simulink model "Control_planta_no_lineal_y_NN_mejor"  (R2023b)
settings: Solver=ode45  StartTime=0.0  StopTime=5000  RelTol=1e-3
values from neighbouring files (symbols this model uses):
  D = 0    [control_pid_tuning.m]
libraries: neural x98, simulink x9
(part 1 of 5)
settings Model: Creator=q  LastModifiedBy=q

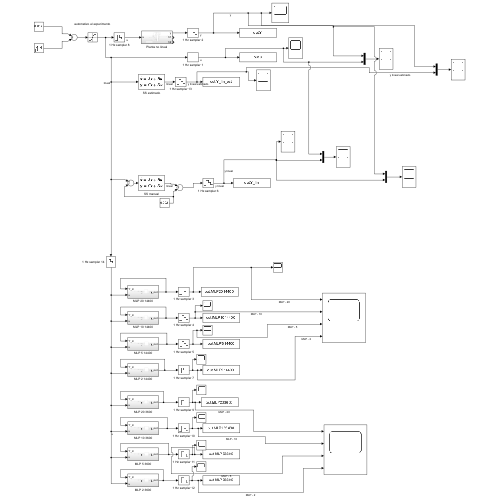
[thumbnail: Simulink's stored preview of the top-level diagram]
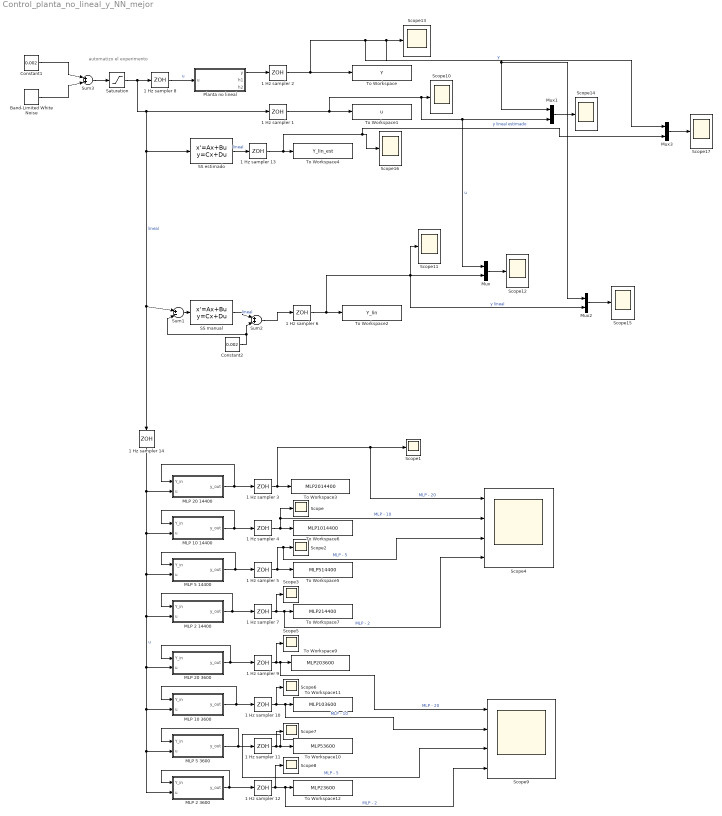
== system Control_planta_no_lineal_y_NN_mejor ==
  note: automatizo el experimento
  1 Hz sampler {1..14} (14 alike) : ZeroOrderHold
  Band-Limited White Noise : simulink/Sources/Band-Limited White Noise  Cov=[0.000002]  Ts=150  seed=[23341]
  Constant1 : Constant  Value=0.002
  Constant2 : Constant  Value=0.002
  MLP 10 14400 : Subsystem
  MLP 10 3600 : Subsystem
  MLP 2 14400 : Subsystem
  MLP 2 3600 : Subsystem
  MLP 20 14400 : Subsystem
  MLP 20 3600 : Subsystem
  MLP 5 14400 : Subsystem
  MLP 5 3600 : Subsystem
  Mux{,1..3} (4 alike) : Mux  Inputs=2
  Planta no lineal : Subsystem
  SS estimado : StateSpace  A=[-0.023375234759513,0.035713459182280;0.016442055191371,-0.031577082096728]  B=[2.537448139699421;-1.771387482474186]  C=[0.008723840649702,0.012539591066566]  D=0  InitialCondition=0
  SS manual : StateSpace  A=[-0.00359 0.000359;0.00976 -0.04878 ];  B=[2.92; 0]  C=[0 0.004905]  D=0  InitialCondition=0
  Saturation : Saturate  UpperLimit=0.0022  LowerLimit=0.0018
  Scope{,1..3,5..8,10..17} (16 alike) : Scope
  Scope4 : Scope  NumInputPorts=4
  Scope9 : Scope  NumInputPorts=4
  Sum1 : Sum  Inputs=|+-|
  Sum2 : Sum  Inputs=|++|
  Sum3 : Sum  Inputs=|++|
  To Workspace : ToWorkspace  VariableName=Y  SampleTime=1
  To Workspace1 : ToWorkspace  VariableName=u  SampleTime=1
  To Workspace10 : ToWorkspace  VariableName=MLP53600  SampleTime=1
  To Workspace11 : ToWorkspace  VariableName=MLP103600  SampleTime=1
  To Workspace12 : ToWorkspace  VariableName=MLP23600  SampleTime=1
  To Workspace2 : ToWorkspace  VariableName=Y_lin  SampleTime=1
  To Workspace3 : ToWorkspace  VariableName=MLP2014400  SampleTime=1
  To Workspace4 : ToWorkspace  VariableName=Y_lin_est  SampleTime=1
  To Workspace5 : ToWorkspace  VariableName=MLP514400  SampleTime=1
  To Workspace6 : ToWorkspace  VariableName=MLP1014400  SampleTime=1
  To Workspace7 : ToWorkspace  VariableName=MLP214400  SampleTime=1
  To Workspace9 : ToWorkspace  VariableName=MLP203600  SampleTime=1
  wires:
  Planta no lineal/1(y) -> 1 Hz sampler 2/1
  Constant1/1 -> Sum3/1
  Sum3/1 -> Saturation/1
  Band-Limited White Noise/1 -> Sum3/2
  1 Hz sampler 2/1 -> Mux3/1, Mux2/1, Mux1/1, Scope13/1, To Workspace/1  "y"
  1 Hz sampler 1/1 -> Mux1/2, Mux/1, Scope10/1, To Workspace1/1  "u"
  MLP 20 14400/1(y_out) -> 1 Hz sampler 3/1, MLP 20 14400/1(Y_in)
  1 Hz sampler 6/1 -> Mux/2, Mux2/2, Scope11/1, To Workspace2/1  "y lineal"
  MLP 10 14400/1(y_out) -> 1 Hz sampler 4/1, MLP 10 14400/1(Y_in)
  1 Hz sampler 3/1 -> Scope4/1, Scope1/1, To Workspace3/1  "MLP - 20"
  1 Hz sampler 4/1 -> Scope/1, Scope4/2, To Workspace6/1  "MLP - 10"
  1 Hz sampler 5/1 -> Scope4/3, Scope2/1, To Workspace5/1  "MLP - 5"
  MLP 5 14400/1(y_out) -> MLP 5 14400/1(Y_in), 1 Hz sampler 5/1
  MLP 2 14400/1(y_out) -> MLP 2 14400/1(Y_in), 1 Hz sampler 7/1
  1 Hz sampler 7/1 -> Scope4/4, To Workspace7/1, Scope3/1  "MLP - 2"
  1 Hz sampler 12/1 -> Scope9/4, To Workspace12/1, Scope8/1  "MLP - 2"
  MLP 2 3600/1(y_out) -> MLP 2 3600/1(Y_in), 1 Hz sampler 12/1
  MLP 5 3600/1(y_out) -> MLP 5 3600/1(Y_in), 1 Hz sampler 11/1
  1 Hz sampler 10/1 -> Scope9/2, To Workspace11/1, Scope6/1  "MLP - 10"
  1 Hz sampler 9/1 -> Scope5/1, Scope9/1, To Workspace9/1  "MLP - 20"
  MLP 10 3600/1(y_out) -> MLP 10 3600/1(Y_in), 1 Hz sampler 10/1
  MLP 20 3600/1(y_out) -> MLP 20 3600/1(Y_in), 1 Hz sampler 9/1
  1 Hz sampler 14/1 -> MLP 20 14400/2(u), MLP 10 14400/2(u), MLP 5 14400/2(u), MLP 2 14400/2(u), MLP 20 3600/2(u), MLP 10 3600/2(u), MLP 5 3600/2(u), MLP 2 3600/2(u)  "u"
  1 Hz sampler 11/1 -> Scope9/3, To Workspace10/1, Scope7/1  "MLP - 5"
  Mux/1 -> Scope12/1
  Mux1/1 -> Scope14/1
  1 Hz sampler 8/1 -> Planta no lineal/1(u)  "u"
  SS manual/1 -> Sum2/1  "lineal"
  Sum2/1 -> 1 Hz sampler 6/1
  Mux2/1 -> Scope15/1
  SS estimado/1 -> 1 Hz sampler 13/1  "lineal"
  1 Hz sampler 13/1 -> Mux3/2, Scope16/1, To Workspace4/1  "y lineal estimado"
  Mux3/1 -> Scope17/1
  Constant2/1 -> Sum1/2, Sum2/2
  Saturation/1 -> 1 Hz sampler 8/1, 1 Hz sampler 14/1, Sum1/1, SS estimado/1, 1 Hz sampler 1/1  "lineal"
  Sum1/1 -> SS manual/1

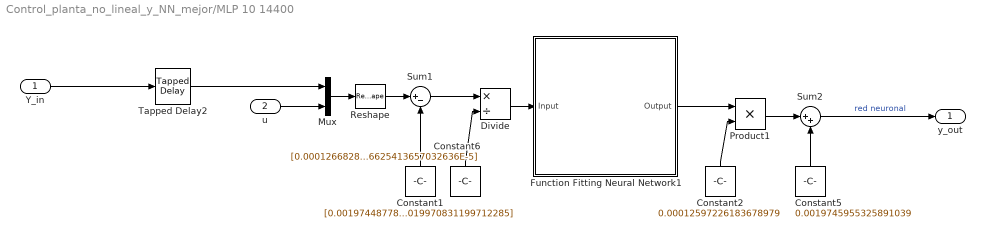
== system Control_planta_no_lineal_y_NN_mejor/MLP 10 14400 ==
  Y_in : Inport
  u : Inport  Port=2
  Constant1 : Constant  Value=[0.0019744877864955233 0.0019743785760481442 0.0019742678131102346 0.0019741553938777768 0.0019740411934791703 0.0019739250574736843 0.0019738067874396224 0.0019736861138403856 0.00197356263591298 0.001973435642133088 0.0019970831199712285]
  Constant2 : Constant  Value=0.00012597226183678979
  Constant5 : Constant  Value=0.0019745955325891039
  Constant6 : Constant  Value=[0.00012668289302772729 0.00012740789305343644 0.00012814838489358016 0.00012890570893586031 0.00012968150046382938 0.00013047781235730809 0.0001312973242993894 0.00013214373888773625 0.00013302266386210407 0.00013394425943220802 9.6625413657032636E-5]
  Divide : Product  Inputs=*/
  Function Fitting Neural Network1 : Subsystem
      mask help: Function Fitting Neural Network
      mask Display: e = 0.06;c1 = [120 150 230]/255;c2 = ([120 150 230]+0)/383;c3 = ([120 150 230]+128)/383;patch([0 1 1 0],[0 0 1 1],c1);patch([0 1 1 1-e 1-e 0+e],[0 0 1 1-e 0+e 0+e],c2);patch([0 0 1 1-e 0+e 0+e],[0 1 1 1-e 1-e 0+e],c3);plot([0 1 1 0 0],[0 0 1 1 0]);fprintf('NNET');port_label('input',1,' Input');port_label('output',1,'Output ');
  Mux : Mux  Inputs=2
  Product1 : Product
  Reshape : Reshape  OutputDimensionality=Column vector (2-D)
  Sum1 : Sum  Inputs=|+-
  Sum2 : Sum  Inputs=|++
  Tapped Delay2 : simulink/Discrete/Tapped Delay  vinit=0  samptime=1  NumDelays=10  DelayOrder=Newest  includeCurrent=off
  y_out : Outport
  wires:
  Sum2/1 -> y_out/1  "red neuronal"
  u/1 -> Mux/2
  Y_in/1 -> Tapped Delay2/1
  Sum1/1 -> Divide/1
  Constant2/1 -> Product1/2
  Product1/1 -> Sum2/1
  Constant5/1 -> Sum2/2
  Constant1/1 -> Sum1/2
  Constant6/1 -> Divide/2
  Tapped Delay2/1 -> Mux/1
  Mux/1 -> Reshape/1
  Reshape/1 -> Sum1/1
  Function Fitting Neural Network1/1(Output) -> Product1/1
  Divide/1 -> Function Fitting Neural Network1/1(Input)

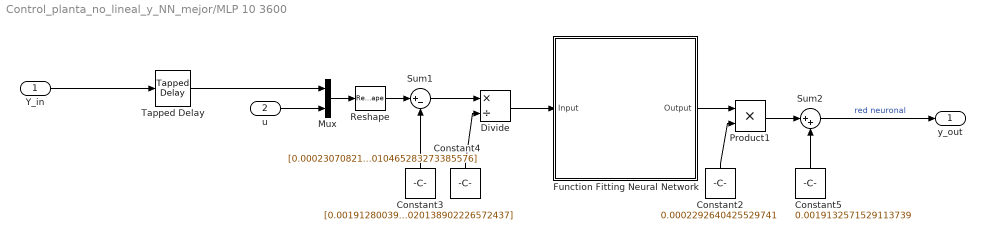
== system Control_planta_no_lineal_y_NN_mejor/MLP 10 3600 ==
  Y_in : Inport
  u : Inport  Port=2
  Constant2 : Constant  Value=0.0002292640425529741
  Constant3 : Constant  Value=[0.0019128003958595781 0.0019123379656579044 0.0019118695096077166 0.0019113946122121862 0.0019109127735299576 0.0019104233750979415 0.0019099256221635427 0.0019094184349221579 0.001908900207568905 0.0019083680886586006 0.0020138902226572437]
  Constant4 : Constant  Value=[0.00023070821663901105 0.00023218152875557362 0.00023368631301103448 0.00023522535857641475 0.00023680207245178661 0.00023842073740024686 0.00024008695208435038 0.00024180846512612068 0.00024359703442975925 0.00024547401204017618 0.00010465283273385576]
  Constant5 : Constant  Value=0.0019132571529113739
  Divide : Product  Inputs=*/
  Function Fitting Neural Network : Subsystem
      mask help: Function Fitting Neural Network
      mask Display: e = 0.06;c1 = [120 150 230]/255;c2 = ([120 150 230]+0)/383;c3 = ([120 150 230]+128)/383;patch([0 1 1 0],[0 0 1 1],c1);patch([0 1 1 1-e 1-e 0+e],[0 0 1 1-e 0+e 0+e],c2);patch([0 0 1 1-e 0+e 0+e],[0 1 1 1-e 1-e 0+e],c3);plot([0 1 1 0 0],[0 0 1 1 0]);fprintf('NNET');port_label('input',1,' Input');port_label('output',1,'Output ');
  Mux : Mux  Inputs=2
  Product1 : Product
  Reshape : Reshape  OutputDimensionality=Column vector (2-D)
  Sum1 : Sum  Inputs=|+-
  Sum2 : Sum  Inputs=|++
  Tapped Delay : simulink/Discrete/Tapped Delay  vinit=0  samptime=-1  NumDelays=10  DelayOrder=Newest  includeCurrent=off
  y_out : Outport
  wires:
  Constant4/1 -> Divide/2
  Mux/1 -> Reshape/1
  Tapped Delay/1 -> Mux/1
  Reshape/1 -> Sum1/1
  Product1/1 -> Sum2/1
  Sum2/1 -> y_out/1  "red neuronal"
  Constant5/1 -> Sum2/2
  Sum1/1 -> Divide/1
  u/1 -> Mux/2
  Constant2/1 -> Product1/2
  Constant3/1 -> Sum1/2
  Function Fitting Neural Network/1(Output) -> Product1/1
  Y_in/1 -> Tapped Delay/1
  Divide/1 -> Function Fitting Neural Network/1(Input)

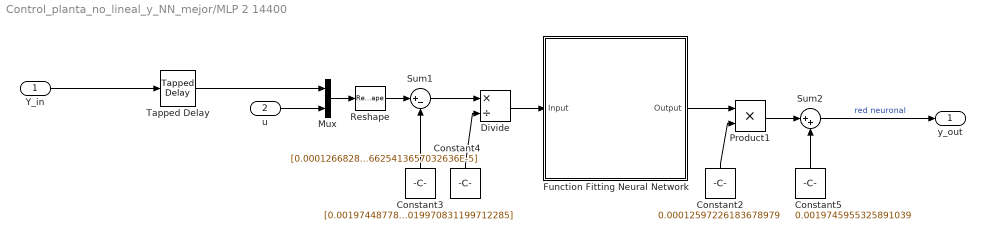
== system Control_planta_no_lineal_y_NN_mejor/MLP 2 14400 ==
  Y_in : Inport
  u : Inport  Port=2
  Constant2 : Constant  Value=0.00012597226183678979
  Constant3 : Constant  Value=[0.0019744877864955233 0.0019743785760481442 0.0019742678131102346 0.0019741553938777768 0.0019740411934791703 0.0019739250574736843 0.0019738067874396224 0.0019736861138403856 0.00197356263591298 0.001973435642133088 0.0019970831199712285]
  Constant4 : Constant  Value=[0.00012668289302772729 0.00012740789305343644 0.00012814838489358016 0.00012890570893586031 0.00012968150046382938 0.00013047781235730809 0.0001312973242993894 0.00013214373888773625 0.00013302266386210407 0.00013394425943220802 9.6625413657032636E-5]
  Constant5 : Constant  Value=0.0019745955325891039
  Divide : Product  Inputs=*/
  Function Fitting Neural Network : Subsystem
      mask help: Function Fitting Neural Network
      mask Display: e = 0.06;c1 = [120 150 230]/255;c2 = ([120 150 230]+0)/383;c3 = ([120 150 230]+128)/383;patch([0 1 1 0],[0 0 1 1],c1);patch([0 1 1 1-e 1-e 0+e],[0 0 1 1-e 0+e 0+e],c2);patch([0 0 1 1-e 0+e 0+e],[0 1 1 1-e 1-e 0+e],c3);plot([0 1 1 0 0],[0 0 1 1 0]);fprintf('NNET');port_label('input',1,' Input');port_label('output',1,'Output ');
  Mux : Mux  Inputs=2
  Product1 : Product
  Reshape : Reshape  OutputDimensionality=Column vector (2-D)
  Sum1 : Sum  Inputs=|+-
  Sum2 : Sum  Inputs=|++
  Tapped Delay : simulink/Discrete/Tapped Delay  vinit=0  samptime=-1  NumDelays=10  DelayOrder=Newest  includeCurrent=off
  y_out : Outport
  wires:
  Sum2/1 -> y_out/1  "red neuronal"
  u/1 -> Mux/2
  Y_in/1 -> Tapped Delay/1
  Sum1/1 -> Divide/1
  Constant2/1 -> Product1/2
  Product1/1 -> Sum2/1
  Constant5/1 -> Sum2/2
  Constant3/1 -> Sum1/2
  Constant4/1 -> Divide/2
  Mux/1 -> Reshape/1
  Reshape/1 -> Sum1/1
  Tapped Delay/1 -> Mux/1
  Divide/1 -> Function Fitting Neural Network/1(Input)
  Function Fitting Neural Network/1(Output) -> Product1/1

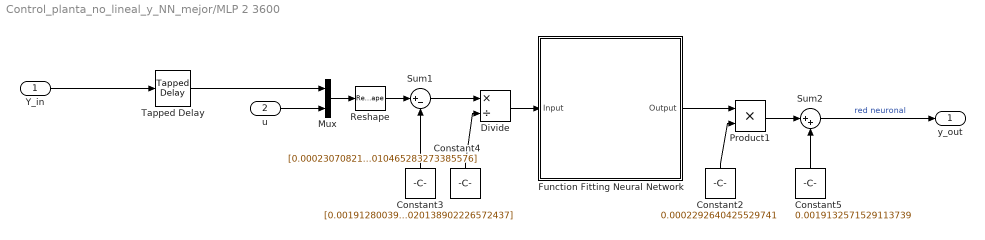
== system Control_planta_no_lineal_y_NN_mejor/MLP 2 3600 ==
  Y_in : Inport
  u : Inport  Port=2
  Constant2 : Constant  Value=0.0002292640425529741
  Constant3 : Constant  Value=[0.0019128003958595781 0.0019123379656579044 0.0019118695096077166 0.0019113946122121862 0.0019109127735299576 0.0019104233750979415 0.0019099256221635427 0.0019094184349221579 0.001908900207568905 0.0019083680886586006 0.0020138902226572437]
  Constant4 : Constant  Value=[0.00023070821663901105 0.00023218152875557362 0.00023368631301103448 0.00023522535857641475 0.00023680207245178661 0.00023842073740024686 0.00024008695208435038 0.00024180846512612068 0.00024359703442975925 0.00024547401204017618 0.00010465283273385576]
  Constant5 : Constant  Value=0.0019132571529113739
  Divide : Product  Inputs=*/
  Function Fitting Neural Network : Subsystem
      mask help: Function Fitting Neural Network
      mask Display: e = 0.06;c1 = [120 150 230]/255;c2 = ([120 150 230]+0)/383;c3 = ([120 150 230]+128)/383;patch([0 1 1 0],[0 0 1 1],c1);patch([0 1 1 1-e 1-e 0+e],[0 0 1 1-e 0+e 0+e],c2);patch([0 0 1 1-e 0+e 0+e],[0 1 1 1-e 1-e 0+e],c3);plot([0 1 1 0 0],[0 0 1 1 0]);fprintf('NNET');port_label('input',1,' Input');port_label('output',1,'Output ');
  Mux : Mux  Inputs=2
  Product1 : Product
  Reshape : Reshape  OutputDimensionality=Column vector (2-D)
  Sum1 : Sum  Inputs=|+-
  Sum2 : Sum  Inputs=|++
  Tapped Delay : simulink/Discrete/Tapped Delay  vinit=0  samptime=-1  NumDelays=10  DelayOrder=Newest  includeCurrent=off
  y_out : Outport
  wires:
  Constant4/1 -> Divide/2
  Mux/1 -> Reshape/1
  Tapped Delay/1 -> Mux/1
  Reshape/1 -> Sum1/1
  Product1/1 -> Sum2/1
  Sum2/1 -> y_out/1  "red neuronal"
  Constant5/1 -> Sum2/2
  Sum1/1 -> Divide/1
  u/1 -> Mux/2
  Constant2/1 -> Product1/2
  Constant3/1 -> Sum1/2
  Function Fitting Neural Network/1(Output) -> Product1/1
  Y_in/1 -> Tapped Delay/1
  Divide/1 -> Function Fitting Neural Network/1(Input)

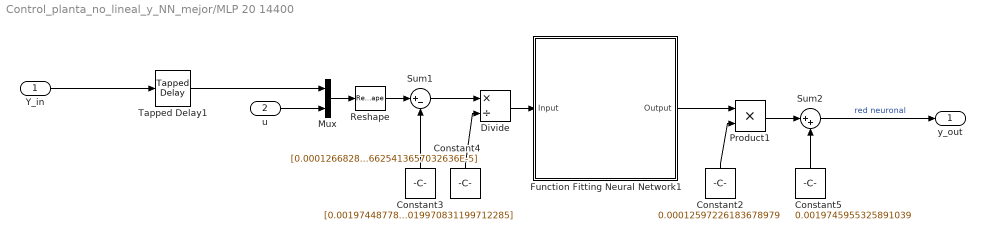
== system Control_planta_no_lineal_y_NN_mejor/MLP 20 14400 ==
  Y_in : Inport
  u : Inport  Port=2
  Constant2 : Constant  Value=0.00012597226183678979
  Constant3 : Constant  Value=[0.0019744877864955233 0.0019743785760481442 0.0019742678131102346 0.0019741553938777768 0.0019740411934791703 0.0019739250574736843 0.0019738067874396224 0.0019736861138403856 0.00197356263591298 0.001973435642133088 0.0019970831199712285]
  Constant4 : Constant  Value=[0.00012668289302772729 0.00012740789305343644 0.00012814838489358016 0.00012890570893586031 0.00012968150046382938 0.00013047781235730809 0.0001312973242993894 0.00013214373888773625 0.00013302266386210407 0.00013394425943220802 9.6625413657032636E-5]
  Constant5 : Constant  Value=0.0019745955325891039
  Divide : Product  Inputs=*/
  Function Fitting Neural Network1 : Subsystem
      mask help: Function Fitting Neural Network
      mask Display: e = 0.06;c1 = [120 150 230]/255;c2 = ([120 150 230]+0)/383;c3 = ([120 150 230]+128)/383;patch([0 1 1 0],[0 0 1 1],c1);patch([0 1 1 1-e 1-e 0+e],[0 0 1 1-e 0+e 0+e],c2);patch([0 0 1 1-e 0+e 0+e],[0 1 1 1-e 1-e 0+e],c3);plot([0 1 1 0 0],[0 0 1 1 0]);fprintf('NNET');port_label('input',1,' Input');port_label('output',1,'Output ');
  Mux : Mux  Inputs=2
  Product1 : Product
  Reshape : Reshape  OutputDimensionality=Column vector (2-D)
  Sum1 : Sum  Inputs=|+-
  Sum2 : Sum  Inputs=|++
  Tapped Delay1 : simulink/Discrete/Tapped Delay  vinit=0  samptime=1  NumDelays=10  DelayOrder=Newest  includeCurrent=off
  y_out : Outport
  wires:
  Constant3/1 -> Sum1/2
  Constant4/1 -> Divide/2
  Mux/1 -> Reshape/1
  Tapped Delay1/1 -> Mux/1
  Sum1/1 -> Divide/1
  Constant5/1 -> Sum2/2
  Reshape/1 -> Sum1/1
  Product1/1 -> Sum2/1
  Constant2/1 -> Product1/2
  Y_in/1 -> Tapped Delay1/1
  u/1 -> Mux/2
  Sum2/1 -> y_out/1  "red neuronal"
  Divide/1 -> Function Fitting Neural Network1/1(Input)
  Function Fitting Neural Network1/1(Output) -> Product1/1

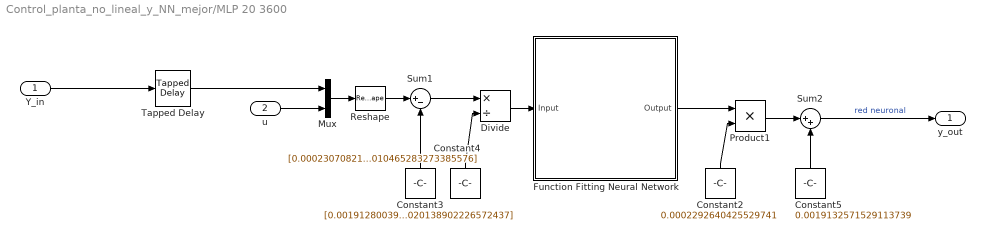
== system Control_planta_no_lineal_y_NN_mejor/MLP 20 3600 ==
  Y_in : Inport
  u : Inport  Port=2
  Constant2 : Constant  Value=0.0002292640425529741
  Constant3 : Constant  Value=[0.0019128003958595781 0.0019123379656579044 0.0019118695096077166 0.0019113946122121862 0.0019109127735299576 0.0019104233750979415 0.0019099256221635427 0.0019094184349221579 0.001908900207568905 0.0019083680886586006 0.0020138902226572437]
  Constant4 : Constant  Value=[0.00023070821663901105 0.00023218152875557362 0.00023368631301103448 0.00023522535857641475 0.00023680207245178661 0.00023842073740024686 0.00024008695208435038 0.00024180846512612068 0.00024359703442975925 0.00024547401204017618 0.00010465283273385576]
  Constant5 : Constant  Value=0.0019132571529113739
  Divide : Product  Inputs=*/
  Function Fitting Neural Network : Subsystem
      mask help: Function Fitting Neural Network
      mask Display: e = 0.06;c1 = [120 150 230]/255;c2 = ([120 150 230]+0)/383;c3 = ([120 150 230]+128)/383;patch([0 1 1 0],[0 0 1 1],c1);patch([0 1 1 1-e 1-e 0+e],[0 0 1 1-e 0+e 0+e],c2);patch([0 0 1 1-e 0+e 0+e],[0 1 1 1-e 1-e 0+e],c3);plot([0 1 1 0 0],[0 0 1 1 0]);fprintf('NNET');port_label('input',1,' Input');port_label('output',1,'Output ');
  Mux : Mux  Inputs=2
  Product1 : Product
  Reshape : Reshape  OutputDimensionality=Column vector (2-D)
  Sum1 : Sum  Inputs=|+-
  Sum2 : Sum  Inputs=|++
  Tapped Delay : simulink/Discrete/Tapped Delay  vinit=0  samptime=-1  NumDelays=10  DelayOrder=Newest  includeCurrent=off
  y_out : Outport
  wires:
  Sum2/1 -> y_out/1  "red neuronal"
  u/1 -> Mux/2
  Y_in/1 -> Tapped Delay/1
  Sum1/1 -> Divide/1
  Constant2/1 -> Product1/2
  Product1/1 -> Sum2/1
  Constant5/1 -> Sum2/2
  Constant3/1 -> Sum1/2
  Constant4/1 -> Divide/2
  Tapped Delay/1 -> Mux/1
  Mux/1 -> Reshape/1
  Reshape/1 -> Sum1/1
  Function Fitting Neural Network/1(Output) -> Product1/1
  Divide/1 -> Function Fitting Neural Network/1(Input)

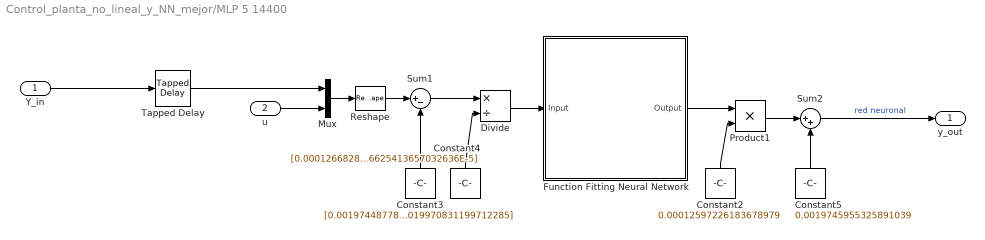
== system Control_planta_no_lineal_y_NN_mejor/MLP 5 14400 ==
  Y_in : Inport
  u : Inport  Port=2
  Constant2 : Constant  Value=0.00012597226183678979
  Constant3 : Constant  Value=[0.0019744877864955233 0.0019743785760481442 0.0019742678131102346 0.0019741553938777768 0.0019740411934791703 0.0019739250574736843 0.0019738067874396224 0.0019736861138403856 0.00197356263591298 0.001973435642133088 0.0019970831199712285]
  Constant4 : Constant  Value=[0.00012668289302772729 0.00012740789305343644 0.00012814838489358016 0.00012890570893586031 0.00012968150046382938 0.00013047781235730809 0.0001312973242993894 0.00013214373888773625 0.00013302266386210407 0.00013394425943220802 9.6625413657032636E-5]
  Constant5 : Constant  Value=0.0019745955325891039
  Divide : Product  Inputs=*/
  Function Fitting Neural Network : Subsystem
      mask help: Function Fitting Neural Network
      mask Display: e = 0.06;c1 = [120 150 230]/255;c2 = ([120 150 230]+0)/383;c3 = ([120 150 230]+128)/383;patch([0 1 1 0],[0 0 1 1],c1);patch([0 1 1 1-e 1-e 0+e],[0 0 1 1-e 0+e 0+e],c2);patch([0 0 1 1-e 0+e 0+e],[0 1 1 1-e 1-e 0+e],c3);plot([0 1 1 0 0],[0 0 1 1 0]);fprintf('NNET');port_label('input',1,' Input');port_label('output',1,'Output ');
  Mux : Mux  Inputs=2
  Product1 : Product
  Reshape : Reshape  OutputDimensionality=Column vector (2-D)
  Sum1 : Sum  Inputs=|+-
  Sum2 : Sum  Inputs=|++
  Tapped Delay : simulink/Discrete/Tapped Delay  vinit=0  samptime=-1  NumDelays=10  DelayOrder=Newest  includeCurrent=off
  y_out : Outport
  wires:
  Sum2/1 -> y_out/1  "red neuronal"
  u/1 -> Mux/2
  Y_in/1 -> Tapped Delay/1
  Sum1/1 -> Divide/1
  Constant2/1 -> Product1/2
  Product1/1 -> Sum2/1
  Constant5/1 -> Sum2/2
  Constant3/1 -> Sum1/2
  Constant4/1 -> Divide/2
  Tapped Delay/1 -> Mux/1
  Mux/1 -> Reshape/1
  Reshape/1 -> Sum1/1
  Divide/1 -> Function Fitting Neural Network/1(Input)
  Function Fitting Neural Network/1(Output) -> Product1/1

== system Control_planta_no_lineal_y_NN_mejor/MLP 5 3600 ==
  Y_in : Inport
  u : Inport  Port=2
  Constant2 : Constant  Value=0.0002292640425529741
  Constant3 : Constant  Value=[0.0019128003958595781 0.0019123379656579044 0.0019118695096077166 0.0019113946122121862 0.0019109127735299576 0.0019104233750979415 0.0019099256221635427 0.0019094184349221579 0.001908900207568905 0.0019083680886586006 0.0020138902226572437]
  Constant4 : Constant  Value=[0.00023070821663901105 0.00023218152875557362 0.00023368631301103448 0.00023522535857641475 0.00023680207245178661 0.00023842073740024686 0.00024008695208435038 0.00024180846512612068 0.00024359703442975925 0.00024547401204017618 0.00010465283273385576]
  Constant5 : Constant  Value=0.0019132571529113739
  Divide : Product  Inputs=*/
  Function Fitting Neural Network : Subsystem
      mask help: Function Fitting Neural Network
      mask Display: e = 0.06;c1 = [120 150 230]/255;c2 = ([120 150 230]+0)/383;c3 = ([120 150 230]+128)/383;patch([0 1 1 0],[0 0 1 1],c1);patch([0 1 1 1-e 1-e 0+e],[0 0 1 1-e 0+e 0+e],c2);patch([0 0 1 1-e 0+e 0+e],[0 1 1 1-e 1-e 0+e],c3);plot([0 1 1 0 0],[0 0 1 1 0]);fprintf('NNET');port_label('input',1,' Input');port_label('output',1,'Output ');
  Mux : Mux  Inputs=2
  Product1 : Product
  Reshape : Reshape  OutputDimensionality=Column vector (2-D)
  Sum1 : Sum  Inputs=|+-
  Sum2 : Sum  Inputs=|++
  Tapped Delay : simulink/Discrete/Tapped Delay  vinit=0  samptime=-1  NumDelays=10  DelayOrder=Newest  includeCurrent=off
  y_out : Outport
  wires:
  Constant4/1 -> Divide/2
  Mux/1 -> Reshape/1
  Tapped Delay/1 -> Mux/1
  Reshape/1 -> Sum1/1
  Product1/1 -> Sum2/1
  Sum2/1 -> y_out/1  "red neuronal"
  Constant5/1 -> Sum2/2
  Sum1/1 -> Divide/1
  u/1 -> Mux/2
  Constant2/1 -> Product1/2
  Constant3/1 -> Sum1/2
  Y_in/1 -> Tapped Delay/1
  Divide/1 -> Function Fitting Neural Network/1(Input)
  Function Fitting Neural Network/1(Output) -> Product1/1

== system Control_planta_no_lineal_y_NN_mejor/Planta no lineal ==
  note: A1 =0.342   m²   (tanque 1 ≈ 66 cm de diámetro)
      | A2 = 0.126   m²   (tanque 2 ≈ 40 cm diámetro)
  u : Inport
  A1 : Constant  Value=0.342119439975929
  A2 : Constant  Value=0.125663706143592
  Constant1 : Constant  Value=0
  Constant6 : Constant  Value=0
  Integrator1 : Integrator  InitialConditionSource=external
  Integrator2 : Integrator  InitialConditionSource=external
  K12 : Constant  Value=5e-4
  K2 : Constant  Value=1e-3
  MATLAB Function : MATLAB Function  TreatAsAtomicUnit=on
  y : Outport
  h1 : Outport  Port=2
  h2 : Outport  Port=3
  wires:
  K2/1 -> MATLAB Function/5(k2)
  MATLAB Function/3(dh2) -> Integrator2/1
  MATLAB Function/2(dh1) -> Integrator1/1
  Integrator1/1 -> h1/1, MATLAB Function/1(h1)
  Constant6/1 -> Integrator2/2
  A2/1 -> MATLAB Function/7(A2)
  Constant1/1 -> Integrator1/2
  u/1 -> MATLAB Function/3(u)
  MATLAB Function/1(y) -> y/1
  Integrator2/1 -> h2/1, MATLAB Function/2(h2)
  A1/1 -> MATLAB Function/6(A1)
  K12/1 -> MATLAB Function/4(k12)

== system Control_planta_no_lineal_y_NN_mejor/MLP 10 14400/Function Fitting Neural Network1 ==
  Input : Inport  PortDimensions=11
      mask Display: e = 0.06;c1 = [120 230 180]/255;c2 = ([120 230 180]+0)/(256+128);c3 = ([120 230 180]+128)/(256+128);patch([0 1 1 0],[0 0 1 1],c1);patch([0 1 1 1-e 1-e 0+e],[0 0 1 1-e 0+e 0+e],c2);patch([0 0 1 1-e 0+e 0+e],[0 1 1 1-e 1-e 0+e],c3);plot([0 1 1 0 0],[0 0 1 1 0]);
  Layer 1 : Subsystem
      mask Display: e = 0.06;c1 = [120 150 230]/255;c2 = ([120 150 230]+0)/383;c3 = ([120 150 230]+128)/383;patch([0 1 1 0],[0 0 1 1],c1);patch([0 1 1 1-e 1-e 0+e],[0 0 1 1-e 0+e 0+e],c2);patch([0 0 1 1-e 0+e 0+e],[0 1 1 1-e 1-e 0+e],c3);plot([0 1 1 0 0],[0 0 1 1 0]);
  Layer 2 : Subsystem
      mask Display: e = 0.06;c1 = [120 150 230]/255;c2 = ([120 150 230]+0)/383;c3 = ([120 150 230]+128)/383;patch([0 1 1 0],[0 0 1 1],c1);patch([0 1 1 1-e 1-e 0+e],[0 0 1 1-e 0+e 0+e],c2);patch([0 0 1 1-e 0+e 0+e],[0 1 1 1-e 1-e 0+e],c3);plot([0 1 1 0 0],[0 0 1 1 0]);
  Process Input 1 : Subsystem
      mask Display: e = 0.06;c1 = [120 150 230]/255;c2 = ([120 150 230]+0)/383;c3 = ([120 150 230]+128)/383;patch([0 1 1 0],[0 0 1 1],c1);patch([0 1 1 1-e 1-e 0+e],[0 0 1 1-e 0+e 0+e],c2);patch([0 0 1 1-e 0+e 0+e],[0 1 1 1-e 1-e 0+e],c3);plot([0 1 1 0 0],[0 0 1 1 0]);
  Process Output 1 : Subsystem
      mask Display: e = 0.06;c1 = [120 150 230]/255;c2 = ([120 150 230]+0)/383;c3 = ([120 150 230]+128)/383;patch([0 1 1 0],[0 0 1 1],c1);patch([0 1 1 1-e 1-e 0+e],[0 0 1 1-e 0+e 0+e],c2);patch([0 0 1 1-e 0+e 0+e],[0 1 1 1-e 1-e 0+e],c3);plot([0 1 1 0 0],[0 0 1 1 0]);
  Output : Outport  InitialOutput=0
      mask Display: e = 0.06;c1 = [120 230 180]/255;c2 = ([120 230 180]+0)/(256+128);c3 = ([120 230 180]+128)/(256+128);patch([0 1 1 0],[0 0 1 1],c1);patch([0 1 1 1-e 1-e 0+e],[0 0 1 1-e 0+e 0+e],c2);patch([0 0 1 1-e 0+e 0+e],[0 1 1 1-e 1-e 0+e],c3);plot([0 1 1 0 0],[0 0 1 1 0]);
  wires:
  Input/1 -> Process Input 1/1(x)
  Process Output 1/1(y) -> Output/1
  Process Input 1/1(p) -> Layer 1/1("p{1}")
  Layer 1/1("a{1}") -> [feedback1]
  [feedback1] -> Layer 2/1("a{1} ")
  Layer 2/1("a{2}") -> Process Output 1/1(a)

== system Control_planta_no_lineal_y_NN_mejor/MLP 10 3600/Function Fitting Neural Network ==
  Input : Inport  PortDimensions=11
      mask Display: e = 0.06;c1 = [120 230 180]/255;c2 = ([120 230 180]+0)/(256+128);c3 = ([120 230 180]+128)/(256+128);patch([0 1 1 0],[0 0 1 1],c1);patch([0 1 1 1-e 1-e 0+e],[0 0 1 1-e 0+e 0+e],c2);patch([0 0 1 1-e 0+e 0+e],[0 1 1 1-e 1-e 0+e],c3);plot([0 1 1 0 0],[0 0 1 1 0]);
  Layer 1 : Subsystem
      mask Display: e = 0.06;c1 = [120 150 230]/255;c2 = ([120 150 230]+0)/383;c3 = ([120 150 230]+128)/383;patch([0 1 1 0],[0 0 1 1],c1);patch([0 1 1 1-e 1-e 0+e],[0 0 1 1-e 0+e 0+e],c2);patch([0 0 1 1-e 0+e 0+e],[0 1 1 1-e 1-e 0+e],c3);plot([0 1 1 0 0],[0 0 1 1 0]);
  Layer 2 : Subsystem
      mask Display: e = 0.06;c1 = [120 150 230]/255;c2 = ([120 150 230]+0)/383;c3 = ([120 150 230]+128)/383;patch([0 1 1 0],[0 0 1 1],c1);patch([0 1 1 1-e 1-e 0+e],[0 0 1 1-e 0+e 0+e],c2);patch([0 0 1 1-e 0+e 0+e],[0 1 1 1-e 1-e 0+e],c3);plot([0 1 1 0 0],[0 0 1 1 0]);
  Process Input 1 : Subsystem
      mask Display: e = 0.06;c1 = [120 150 230]/255;c2 = ([120 150 230]+0)/383;c3 = ([120 150 230]+128)/383;patch([0 1 1 0],[0 0 1 1],c1);patch([0 1 1 1-e 1-e 0+e],[0 0 1 1-e 0+e 0+e],c2);patch([0 0 1 1-e 0+e 0+e],[0 1 1 1-e 1-e 0+e],c3);plot([0 1 1 0 0],[0 0 1 1 0]);
  Process Output 1 : Subsystem
      mask Display: e = 0.06;c1 = [120 150 230]/255;c2 = ([120 150 230]+0)/383;c3 = ([120 150 230]+128)/383;patch([0 1 1 0],[0 0 1 1],c1);patch([0 1 1 1-e 1-e 0+e],[0 0 1 1-e 0+e 0+e],c2);patch([0 0 1 1-e 0+e 0+e],[0 1 1 1-e 1-e 0+e],c3);plot([0 1 1 0 0],[0 0 1 1 0]);
  Output : Outport  InitialOutput=0
      mask Display: e = 0.06;c1 = [120 230 180]/255;c2 = ([120 230 180]+0)/(256+128);c3 = ([120 230 180]+128)/(256+128);patch([0 1 1 0],[0 0 1 1],c1);patch([0 1 1 1-e 1-e 0+e],[0 0 1 1-e 0+e 0+e],c2);patch([0 0 1 1-e 0+e 0+e],[0 1 1 1-e 1-e 0+e],c3);plot([0 1 1 0 0],[0 0 1 1 0]);
  wires:
  Input/1 -> Process Input 1/1(x)
  Process Output 1/1(y) -> Output/1
  Process Input 1/1(p) -> Layer 1/1("p{1}")
  Layer 1/1("a{1}") -> [feedback1]
  [feedback1] -> Layer 2/1("a{1} ")
  Layer 2/1("a{2}") -> Process Output 1/1(a)

== system Control_planta_no_lineal_y_NN_mejor/MLP 2 14400/Function Fitting Neural Network ==
  Input : Inport  PortDimensions=11
      mask Display: e = 0.06;c1 = [120 230 180]/255;c2 = ([120 230 180]+0)/(256+128);c3 = ([120 230 180]+128)/(256+128);patch([0 1 1 0],[0 0 1 1],c1);patch([0 1 1 1-e 1-e 0+e],[0 0 1 1-e 0+e 0+e],c2);patch([0 0 1 1-e 0+e 0+e],[0 1 1 1-e 1-e 0+e],c3);plot([0 1 1 0 0],[0 0 1 1 0]);
  Layer 1 : Subsystem
      mask Display: e = 0.06;c1 = [120 150 230]/255;c2 = ([120 150 230]+0)/383;c3 = ([120 150 230]+128)/383;patch([0 1 1 0],[0 0 1 1],c1);patch([0 1 1 1-e 1-e 0+e],[0 0 1 1-e 0+e 0+e],c2);patch([0 0 1 1-e 0+e 0+e],[0 1 1 1-e 1-e 0+e],c3);plot([0 1 1 0 0],[0 0 1 1 0]);
  Layer 2 : Subsystem
      mask Display: e = 0.06;c1 = [120 150 230]/255;c2 = ([120 150 230]+0)/383;c3 = ([120 150 230]+128)/383;patch([0 1 1 0],[0 0 1 1],c1);patch([0 1 1 1-e 1-e 0+e],[0 0 1 1-e 0+e 0+e],c2);patch([0 0 1 1-e 0+e 0+e],[0 1 1 1-e 1-e 0+e],c3);plot([0 1 1 0 0],[0 0 1 1 0]);
  Process Input 1 : Subsystem
      mask Display: e = 0.06;c1 = [120 150 230]/255;c2 = ([120 150 230]+0)/383;c3 = ([120 150 230]+128)/383;patch([0 1 1 0],[0 0 1 1],c1);patch([0 1 1 1-e 1-e 0+e],[0 0 1 1-e 0+e 0+e],c2);patch([0 0 1 1-e 0+e 0+e],[0 1 1 1-e 1-e 0+e],c3);plot([0 1 1 0 0],[0 0 1 1 0]);
  Process Output 1 : Subsystem
      mask Display: e = 0.06;c1 = [120 150 230]/255;c2 = ([120 150 230]+0)/383;c3 = ([120 150 230]+128)/383;patch([0 1 1 0],[0 0 1 1],c1);patch([0 1 1 1-e 1-e 0+e],[0 0 1 1-e 0+e 0+e],c2);patch([0 0 1 1-e 0+e 0+e],[0 1 1 1-e 1-e 0+e],c3);plot([0 1 1 0 0],[0 0 1 1 0]);
  Output : Outport  InitialOutput=0
      mask Display: e = 0.06;c1 = [120 230 180]/255;c2 = ([120 230 180]+0)/(256+128);c3 = ([120 230 180]+128)/(256+128);patch([0 1 1 0],[0 0 1 1],c1);patch([0 1 1 1-e 1-e 0+e],[0 0 1 1-e 0+e 0+e],c2);patch([0 0 1 1-e 0+e 0+e],[0 1 1 1-e 1-e 0+e],c3);plot([0 1 1 0 0],[0 0 1 1 0]);
  wires:
  Input/1 -> Process Input 1/1(x)
  Process Output 1/1(y) -> Output/1
  Process Input 1/1(p) -> Layer 1/1("p{1}")
  Layer 1/1("a{1}") -> [feedback1]
  [feedback1] -> Layer 2/1("a{1} ")
  Layer 2/1("a{2}") -> Process Output 1/1(a)

== system Control_planta_no_lineal_y_NN_mejor/MLP 2 3600/Function Fitting Neural Network ==
  Input : Inport  PortDimensions=11
      mask Display: e = 0.06;c1 = [120 230 180]/255;c2 = ([120 230 180]+0)/(256+128);c3 = ([120 230 180]+128)/(256+128);patch([0 1 1 0],[0 0 1 1],c1);patch([0 1 1 1-e 1-e 0+e],[0 0 1 1-e 0+e 0+e],c2);patch([0 0 1 1-e 0+e 0+e],[0 1 1 1-e 1-e 0+e],c3);plot([0 1 1 0 0],[0 0 1 1 0]);
  Layer 1 : Subsystem
      mask Display: e = 0.06;c1 = [120 150 230]/255;c2 = ([120 150 230]+0)/383;c3 = ([120 150 230]+128)/383;patch([0 1 1 0],[0 0 1 1],c1);patch([0 1 1 1-e 1-e 0+e],[0 0 1 1-e 0+e 0+e],c2);patch([0 0 1 1-e 0+e 0+e],[0 1 1 1-e 1-e 0+e],c3);plot([0 1 1 0 0],[0 0 1 1 0]);
  Layer 2 : Subsystem
      mask Display: e = 0.06;c1 = [120 150 230]/255;c2 = ([120 150 230]+0)/383;c3 = ([120 150 230]+128)/383;patch([0 1 1 0],[0 0 1 1],c1);patch([0 1 1 1-e 1-e 0+e],[0 0 1 1-e 0+e 0+e],c2);patch([0 0 1 1-e 0+e 0+e],[0 1 1 1-e 1-e 0+e],c3);plot([0 1 1 0 0],[0 0 1 1 0]);
  Process Input 1 : Subsystem
      mask Display: e = 0.06;c1 = [120 150 230]/255;c2 = ([120 150 230]+0)/383;c3 = ([120 150 230]+128)/383;patch([0 1 1 0],[0 0 1 1],c1);patch([0 1 1 1-e 1-e 0+e],[0 0 1 1-e 0+e 0+e],c2);patch([0 0 1 1-e 0+e 0+e],[0 1 1 1-e 1-e 0+e],c3);plot([0 1 1 0 0],[0 0 1 1 0]);
  Process Output 1 : Subsystem
      mask Display: e = 0.06;c1 = [120 150 230]/255;c2 = ([120 150 230]+0)/383;c3 = ([120 150 230]+128)/383;patch([0 1 1 0],[0 0 1 1],c1);patch([0 1 1 1-e 1-e 0+e],[0 0 1 1-e 0+e 0+e],c2);patch([0 0 1 1-e 0+e 0+e],[0 1 1 1-e 1-e 0+e],c3);plot([0 1 1 0 0],[0 0 1 1 0]);
  Output : Outport  InitialOutput=0
      mask Display: e = 0.06;c1 = [120 230 180]/255;c2 = ([120 230 180]+0)/(256+128);c3 = ([120 230 180]+128)/(256+128);patch([0 1 1 0],[0 0 1 1],c1);patch([0 1 1 1-e 1-e 0+e],[0 0 1 1-e 0+e 0+e],c2);patch([0 0 1 1-e 0+e 0+e],[0 1 1 1-e 1-e 0+e],c3);plot([0 1 1 0 0],[0 0 1 1 0]);
  wires:
  Input/1 -> Process Input 1/1(x)
  Process Output 1/1(y) -> Output/1
  Process Input 1/1(p) -> Layer 1/1("p{1}")
  Layer 1/1("a{1}") -> [feedback1]
  [feedback1] -> Layer 2/1("a{1} ")
  Layer 2/1("a{2}") -> Process Output 1/1(a)

== system Control_planta_no_lineal_y_NN_mejor/MLP 20 14400/Function Fitting Neural Network1 ==
  Input : Inport  PortDimensions=11
      mask Display: e = 0.06;c1 = [120 230 180]/255;c2 = ([120 230 180]+0)/(256+128);c3 = ([120 230 180]+128)/(256+128);patch([0 1 1 0],[0 0 1 1],c1);patch([0 1 1 1-e 1-e 0+e],[0 0 1 1-e 0+e 0+e],c2);patch([0 0 1 1-e 0+e 0+e],[0 1 1 1-e 1-e 0+e],c3);plot([0 1 1 0 0],[0 0 1 1 0]);
  Layer 1 : Subsystem
      mask Display: e = 0.06;c1 = [120 150 230]/255;c2 = ([120 150 230]+0)/383;c3 = ([120 150 230]+128)/383;patch([0 1 1 0],[0 0 1 1],c1);patch([0 1 1 1-e 1-e 0+e],[0 0 1 1-e 0+e 0+e],c2);patch([0 0 1 1-e 0+e 0+e],[0 1 1 1-e 1-e 0+e],c3);plot([0 1 1 0 0],[0 0 1 1 0]);
  Layer 2 : Subsystem
      mask Display: e = 0.06;c1 = [120 150 230]/255;c2 = ([120 150 230]+0)/383;c3 = ([120 150 230]+128)/383;patch([0 1 1 0],[0 0 1 1],c1);patch([0 1 1 1-e 1-e 0+e],[0 0 1 1-e 0+e 0+e],c2);patch([0 0 1 1-e 0+e 0+e],[0 1 1 1-e 1-e 0+e],c3);plot([0 1 1 0 0],[0 0 1 1 0]);
  Process Input 1 : Subsystem
      mask Display: e = 0.06;c1 = [120 150 230]/255;c2 = ([120 150 230]+0)/383;c3 = ([120 150 230]+128)/383;patch([0 1 1 0],[0 0 1 1],c1);patch([0 1 1 1-e 1-e 0+e],[0 0 1 1-e 0+e 0+e],c2);patch([0 0 1 1-e 0+e 0+e],[0 1 1 1-e 1-e 0+e],c3);plot([0 1 1 0 0],[0 0 1 1 0]);
  Process Output 1 : Subsystem
      mask Display: e = 0.06;c1 = [120 150 230]/255;c2 = ([120 150 230]+0)/383;c3 = ([120 150 230]+128)/383;patch([0 1 1 0],[0 0 1 1],c1);patch([0 1 1 1-e 1-e 0+e],[0 0 1 1-e 0+e 0+e],c2);patch([0 0 1 1-e 0+e 0+e],[0 1 1 1-e 1-e 0+e],c3);plot([0 1 1 0 0],[0 0 1 1 0]);
  Output : Outport  InitialOutput=0
      mask Display: e = 0.06;c1 = [120 230 180]/255;c2 = ([120 230 180]+0)/(256+128);c3 = ([120 230 180]+128)/(256+128);patch([0 1 1 0],[0 0 1 1],c1);patch([0 1 1 1-e 1-e 0+e],[0 0 1 1-e 0+e 0+e],c2);patch([0 0 1 1-e 0+e 0+e],[0 1 1 1-e 1-e 0+e],c3);plot([0 1 1 0 0],[0 0 1 1 0]);
  wires:
  Input/1 -> Process Input 1/1(x)
  Process Output 1/1(y) -> Output/1
  Process Input 1/1(p) -> Layer 1/1("p{1}")
  Layer 1/1("a{1}") -> [feedback1]
  [feedback1] -> Layer 2/1("a{1} ")
  Layer 2/1("a{2}") -> Process Output 1/1(a)

== system Control_planta_no_lineal_y_NN_mejor/MLP 20 3600/Function Fitting Neural Network ==
  Input : Inport  PortDimensions=11
      mask Display: e = 0.06;c1 = [120 230 180]/255;c2 = ([120 230 180]+0)/(256+128);c3 = ([120 230 180]+128)/(256+128);patch([0 1 1 0],[0 0 1 1],c1);patch([0 1 1 1-e 1-e 0+e],[0 0 1 1-e 0+e 0+e],c2);patch([0 0 1 1-e 0+e 0+e],[0 1 1 1-e 1-e 0+e],c3);plot([0 1 1 0 0],[0 0 1 1 0]);
  Layer 1 : Subsystem
      mask Display: e = 0.06;c1 = [120 150 230]/255;c2 = ([120 150 230]+0)/383;c3 = ([120 150 230]+128)/383;patch([0 1 1 0],[0 0 1 1],c1);patch([0 1 1 1-e 1-e 0+e],[0 0 1 1-e 0+e 0+e],c2);patch([0 0 1 1-e 0+e 0+e],[0 1 1 1-e 1-e 0+e],c3);plot([0 1 1 0 0],[0 0 1 1 0]);
  Layer 2 : Subsystem
      mask Display: e = 0.06;c1 = [120 150 230]/255;c2 = ([120 150 230]+0)/383;c3 = ([120 150 230]+128)/383;patch([0 1 1 0],[0 0 1 1],c1);patch([0 1 1 1-e 1-e 0+e],[0 0 1 1-e 0+e 0+e],c2);patch([0 0 1 1-e 0+e 0+e],[0 1 1 1-e 1-e 0+e],c3);plot([0 1 1 0 0],[0 0 1 1 0]);
  Process Input 1 : Subsystem
      mask Display: e = 0.06;c1 = [120 150 230]/255;c2 = ([120 150 230]+0)/383;c3 = ([120 150 230]+128)/383;patch([0 1 1 0],[0 0 1 1],c1);patch([0 1 1 1-e 1-e 0+e],[0 0 1 1-e 0+e 0+e],c2);patch([0 0 1 1-e 0+e 0+e],[0 1 1 1-e 1-e 0+e],c3);plot([0 1 1 0 0],[0 0 1 1 0]);
  Process Output 1 : Subsystem
      mask Display: e = 0.06;c1 = [120 150 230]/255;c2 = ([120 150 230]+0)/383;c3 = ([120 150 230]+128)/383;patch([0 1 1 0],[0 0 1 1],c1);patch([0 1 1 1-e 1-e 0+e],[0 0 1 1-e 0+e 0+e],c2);patch([0 0 1 1-e 0+e 0+e],[0 1 1 1-e 1-e 0+e],c3);plot([0 1 1 0 0],[0 0 1 1 0]);
  Output : Outport  InitialOutput=0
      mask Display: e = 0.06;c1 = [120 230 180]/255;c2 = ([120 230 180]+0)/(256+128);c3 = ([120 230 180]+128)/(256+128);patch([0 1 1 0],[0 0 1 1],c1);patch([0 1 1 1-e 1-e 0+e],[0 0 1 1-e 0+e 0+e],c2);patch([0 0 1 1-e 0+e 0+e],[0 1 1 1-e 1-e 0+e],c3);plot([0 1 1 0 0],[0 0 1 1 0]);
  wires:
  Input/1 -> Process Input 1/1(x)
  Process Output 1/1(y) -> Output/1
  Process Input 1/1(p) -> Layer 1/1("p{1}")
  Layer 1/1("a{1}") -> [feedback1]
  [feedback1] -> Layer 2/1("a{1} ")
  Layer 2/1("a{2}") -> Process Output 1/1(a)

== system Control_planta_no_lineal_y_NN_mejor/MLP 5 14400/Function Fitting Neural Network ==
  Input : Inport  PortDimensions=11
      mask Display: e = 0.06;c1 = [120 230 180]/255;c2 = ([120 230 180]+0)/(256+128);c3 = ([120 230 180]+128)/(256+128);patch([0 1 1 0],[0 0 1 1],c1);patch([0 1 1 1-e 1-e 0+e],[0 0 1 1-e 0+e 0+e],c2);patch([0 0 1 1-e 0+e 0+e],[0 1 1 1-e 1-e 0+e],c3);plot([0 1 1 0 0],[0 0 1 1 0]);
  Layer 1 : Subsystem
      mask Display: e = 0.06;c1 = [120 150 230]/255;c2 = ([120 150 230]+0)/383;c3 = ([120 150 230]+128)/383;patch([0 1 1 0],[0 0 1 1],c1);patch([0 1 1 1-e 1-e 0+e],[0 0 1 1-e 0+e 0+e],c2);patch([0 0 1 1-e 0+e 0+e],[0 1 1 1-e 1-e 0+e],c3);plot([0 1 1 0 0],[0 0 1 1 0]);
  Layer 2 : Subsystem
      mask Display: e = 0.06;c1 = [120 150 230]/255;c2 = ([120 150 230]+0)/383;c3 = ([120 150 230]+128)/383;patch([0 1 1 0],[0 0 1 1],c1);patch([0 1 1 1-e 1-e 0+e],[0 0 1 1-e 0+e 0+e],c2);patch([0 0 1 1-e 0+e 0+e],[0 1 1 1-e 1-e 0+e],c3);plot([0 1 1 0 0],[0 0 1 1 0]);
  Process Input 1 : Subsystem
      mask Display: e = 0.06;c1 = [120 150 230]/255;c2 = ([120 150 230]+0)/383;c3 = ([120 150 230]+128)/383;patch([0 1 1 0],[0 0 1 1],c1);patch([0 1 1 1-e 1-e 0+e],[0 0 1 1-e 0+e 0+e],c2);patch([0 0 1 1-e 0+e 0+e],[0 1 1 1-e 1-e 0+e],c3);plot([0 1 1 0 0],[0 0 1 1 0]);
  Process Output 1 : Subsystem
      mask Display: e = 0.06;c1 = [120 150 230]/255;c2 = ([120 150 230]+0)/383;c3 = ([120 150 230]+128)/383;patch([0 1 1 0],[0 0 1 1],c1);patch([0 1 1 1-e 1-e 0+e],[0 0 1 1-e 0+e 0+e],c2);patch([0 0 1 1-e 0+e 0+e],[0 1 1 1-e 1-e 0+e],c3);plot([0 1 1 0 0],[0 0 1 1 0]);
  Output : Outport  InitialOutput=0
      mask Display: e = 0.06;c1 = [120 230 180]/255;c2 = ([120 230 180]+0)/(256+128);c3 = ([120 230 180]+128)/(256+128);patch([0 1 1 0],[0 0 1 1],c1);patch([0 1 1 1-e 1-e 0+e],[0 0 1 1-e 0+e 0+e],c2);patch([0 0 1 1-e 0+e 0+e],[0 1 1 1-e 1-e 0+e],c3);plot([0 1 1 0 0],[0 0 1 1 0]);
  wires:
  Input/1 -> Process Input 1/1(x)
  Process Output 1/1(y) -> Output/1
  Process Input 1/1(p) -> Layer 1/1("p{1}")
  Layer 1/1("a{1}") -> [feedback1]
  [feedback1] -> Layer 2/1("a{1} ")
  Layer 2/1("a{2}") -> Process Output 1/1(a)

== system Control_planta_no_lineal_y_NN_mejor/MLP 5 3600/Function Fitting Neural Network ==
  Input : Inport  PortDimensions=11
      mask Display: e = 0.06;c1 = [120 230 180]/255;c2 = ([120 230 180]+0)/(256+128);c3 = ([120 230 180]+128)/(256+128);patch([0 1 1 0],[0 0 1 1],c1);patch([0 1 1 1-e 1-e 0+e],[0 0 1 1-e 0+e 0+e],c2);patch([0 0 1 1-e 0+e 0+e],[0 1 1 1-e 1-e 0+e],c3);plot([0 1 1 0 0],[0 0 1 1 0]);
  Layer 1 : Subsystem
      mask Display: e = 0.06;c1 = [120 150 230]/255;c2 = ([120 150 230]+0)/383;c3 = ([120 150 230]+128)/383;patch([0 1 1 0],[0 0 1 1],c1);patch([0 1 1 1-e 1-e 0+e],[0 0 1 1-e 0+e 0+e],c2);patch([0 0 1 1-e 0+e 0+e],[0 1 1 1-e 1-e 0+e],c3);plot([0 1 1 0 0],[0 0 1 1 0]);
  Layer 2 : Subsystem
      mask Display: e = 0.06;c1 = [120 150 230]/255;c2 = ([120 150 230]+0)/383;c3 = ([120 150 230]+128)/383;patch([0 1 1 0],[0 0 1 1],c1);patch([0 1 1 1-e 1-e 0+e],[0 0 1 1-e 0+e 0+e],c2);patch([0 0 1 1-e 0+e 0+e],[0 1 1 1-e 1-e 0+e],c3);plot([0 1 1 0 0],[0 0 1 1 0]);
  Process Input 1 : Subsystem
      mask Display: e = 0.06;c1 = [120 150 230]/255;c2 = ([120 150 230]+0)/383;c3 = ([120 150 230]+128)/383;patch([0 1 1 0],[0 0 1 1],c1);patch([0 1 1 1-e 1-e 0+e],[0 0 1 1-e 0+e 0+e],c2);patch([0 0 1 1-e 0+e 0+e],[0 1 1 1-e 1-e 0+e],c3);plot([0 1 1 0 0],[0 0 1 1 0]);
  Process Output 1 : Subsystem
      mask Display: e = 0.06;c1 = [120 150 230]/255;c2 = ([120 150 230]+0)/383;c3 = ([120 150 230]+128)/383;patch([0 1 1 0],[0 0 1 1],c1);patch([0 1 1 1-e 1-e 0+e],[0 0 1 1-e 0+e 0+e],c2);patch([0 0 1 1-e 0+e 0+e],[0 1 1 1-e 1-e 0+e],c3);plot([0 1 1 0 0],[0 0 1 1 0]);
  Output : Outport  InitialOutput=0
      mask Display: e = 0.06;c1 = [120 230 180]/255;c2 = ([120 230 180]+0)/(256+128);c3 = ([120 230 180]+128)/(256+128);patch([0 1 1 0],[0 0 1 1],c1);patch([0 1 1 1-e 1-e 0+e],[0 0 1 1-e 0+e 0+e],c2);patch([0 0 1 1-e 0+e 0+e],[0 1 1 1-e 1-e 0+e],c3);plot([0 1 1 0 0],[0 0 1 1 0]);
  wires:
  Input/1 -> Process Input 1/1(x)
  Process Output 1/1(y) -> Output/1
  Process Input 1/1(p) -> Layer 1/1("p{1}")
  Layer 1/1("a{1}") -> [feedback1]
  [feedback1] -> Layer 2/1("a{1} ")
  Layer 2/1("a{2}") -> Process Output 1/1(a)

== system Control_planta_no_lineal_y_NN_mejor/MLP 10 14400/Function Fitting Neural Network1/Layer 1 ==
  "p{1}" : Inport  PortDimensions=11
      mask Display: e = 0.06;c1 = [120 230 180]/255;c2 = ([120 230 180]+0)/(256+128);c3 = ([120 230 180]+128)/(256+128);patch([0 1 1 0],[0 0 1 1],c1);patch([0 1 1 1-e 1-e 0+e],[0 0 1 1-e 0+e 0+e],c2);patch([0 0 1 1-e 0+e 0+e],[0 1 1 1-e 1-e 0+e],c3);plot([0 1 1 0 0],[0 0 1 1 0]);
  Delays 1 : Subsystem
      mask Display: e = 0.06;c1 = [120 150 230]/255;c2 = ([120 150 230]+0)/383;c3 = ([120 150 230]+128)/383;patch([0 1 1 0],[0 0 1 1],c1);patch([0 1 1 1-e 1-e 0+e],[0 0 1 1-e 0+e 0+e],c2);patch([0 0 1 1-e 0+e 0+e],[0 1 1 1-e 1-e 0+e],c3);plot([0 1 1 0 0],[0 0 1 1 0]);disp('0');
  "IW{1,1}" : Subsystem
      mask Display: e = 0.06;c1 = [120 150 230]/255;c2 = ([120 150 230]+0)/383;c3 = ([120 150 230]+128)/383;patch([0 1 1 0],[0 0 1 1],c1);patch([0 1 1 1-e 1-e 0+e],[0 0 1 1-e 0+e 0+e],c2);patch([0 0 1 1-e 0+e 0+e],[0 1 1 1-e 1-e 0+e],c3);plot([0 1 1 0 0],[0 0 1 1 0]);disp('W');
  "b{1}" : Constant  Value=[-0.7485966139215582959565153942094184458255767822265625;0.00984863840066990160748705562809846014715731143951416015625;1.859590875168119605831407170626334846019744873046875;0.280489907628993118127169736908399499952793121337890625;-0.96260096744054468587137307622469961643218994140625;0.8372999391083608689001493985415436327457427978515625;-0.9525263007432152040365735956584103405475616455078125;-3.28214143702767291443933572736568748950958251953125;-3.11908370965059145163422726909630000591278076171875;-1.6882307025306857450885900107095949351787567138671875]
      mask Display: e = 0.06;c1 = [120 150 230]/255;c2 = ([120 150 230]+0)/383;c3 = ([120 150 230]+128)/383;patch([0 1 1 0],[0 0 1 1],c1);patch([0 1 1 1-e 1-e 0+e],[0 0 1 1-e 0+e 0+e],c2);patch([0 0 1 1-e 0+e 0+e],[0 1 1 1-e 1-e 0+e],c3);plot([0 1 1 0 0],[0 0 1 1 0]);disp('b');
  netsum : Sum  Inputs=2  InputSameDT=on  SaturateOnIntegerOverflow=on  OutDataTypeStr=Inherit: Same as first input
      mask Display: e = 0.06;c1 = [120 150 230]/255;c2 = ([120 150 230]+0)/383;c3 = ([120 150 230]+128)/383;patch([0 1 1 0],[0 0 1 1],c1);patch([0 1 1 1-e 1-e 0+e],[0 0 1 1-e 0+e 0+e],c2);patch([0 0 1 1-e 0+e 0+e],[0 1 1 1-e 1-e 0+e],c3);plot([0 1 1 0 0],[0 0 1 1 0]);disp('+');
  tansig : neural/Transfer Functions/tansig
  "a{1}" : Outport  InitialOutput=[0;0;0;0;0;0;0;0;0;0]
      mask Display: e = 0.06;c1 = [120 230 180]/255;c2 = ([120 230 180]+0)/(256+128);c3 = ([120 230 180]+128)/(256+128);patch([0 1 1 0],[0 0 1 1],c1);patch([0 1 1 1-e 1-e 0+e],[0 0 1 1-e 0+e 0+e],c2);patch([0 0 1 1-e 0+e 0+e],[0 1 1 1-e 1-e 0+e],c3);plot([0 1 1 0 0],[0 0 1 1 0]);
  wires:
  "p{1}"/1 -> Delays 1/1("p{1}")
  Delays 1/1("pd{1,1}") -> "IW{1,1}"/1("pd{1,1}")
  "IW{1,1}"/1("iz{1,1}") -> netsum/1
  "b{1}"/1 -> netsum/2
  netsum/1 -> tansig/1
  tansig/1 -> "a{1}"/1

== system Control_planta_no_lineal_y_NN_mejor/MLP 10 14400/Function Fitting Neural Network1/Layer 2 ==
  "a{1} " : Inport  PortDimensions=10
      mask Display: e = 0.06;c1 = [120 230 180]/255;c2 = ([120 230 180]+0)/(256+128);c3 = ([120 230 180]+128)/(256+128);patch([0 1 1 0],[0 0 1 1],c1);patch([0 1 1 1-e 1-e 0+e],[0 0 1 1-e 0+e 0+e],c2);patch([0 0 1 1-e 0+e 0+e],[0 1 1 1-e 1-e 0+e],c3);plot([0 1 1 0 0],[0 0 1 1 0]);
  Delays 1 : Subsystem
      mask Display: e = 0.06;c1 = [120 150 230]/255;c2 = ([120 150 230]+0)/383;c3 = ([120 150 230]+128)/383;patch([0 1 1 0],[0 0 1 1],c1);patch([0 1 1 1-e 1-e 0+e],[0 0 1 1-e 0+e 0+e],c2);patch([0 0 1 1-e 0+e 0+e],[0 1 1 1-e 1-e 0+e],c3);plot([0 1 1 0 0],[0 0 1 1 0]);disp('0');
  "LW{2,1}" : Subsystem
      mask Display: e = 0.06;c1 = [120 150 230]/255;c2 = ([120 150 230]+0)/383;c3 = ([120 150 230]+128)/383;patch([0 1 1 0],[0 0 1 1],c1);patch([0 1 1 1-e 1-e 0+e],[0 0 1 1-e 0+e 0+e],c2);patch([0 0 1 1-e 0+e 0+e],[0 1 1 1-e 1-e 0+e],c3);plot([0 1 1 0 0],[0 0 1 1 0]);disp('W');
  "b{2}" : Constant  Value=-1.743133992428117284845257017877884209156036376953125
      mask Display: e = 0.06;c1 = [120 150 230]/255;c2 = ([120 150 230]+0)/383;c3 = ([120 150 230]+128)/383;patch([0 1 1 0],[0 0 1 1],c1);patch([0 1 1 1-e 1-e 0+e],[0 0 1 1-e 0+e 0+e],c2);patch([0 0 1 1-e 0+e 0+e],[0 1 1 1-e 1-e 0+e],c3);plot([0 1 1 0 0],[0 0 1 1 0]);disp('b');
  netsum : Sum  Inputs=2  InputSameDT=on  SaturateOnIntegerOverflow=on  OutDataTypeStr=Inherit: Same as first input
      mask Display: e = 0.06;c1 = [120 150 230]/255;c2 = ([120 150 230]+0)/383;c3 = ([120 150 230]+128)/383;patch([0 1 1 0],[0 0 1 1],c1);patch([0 1 1 1-e 1-e 0+e],[0 0 1 1-e 0+e 0+e],c2);patch([0 0 1 1-e 0+e 0+e],[0 1 1 1-e 1-e 0+e],c3);plot([0 1 1 0 0],[0 0 1 1 0]);disp('+');
  purelin : neural/Transfer Functions/purelin
  "a{2}" : Outport  InitialOutput=0
      mask Display: e = 0.06;c1 = [120 230 180]/255;c2 = ([120 230 180]+0)/(256+128);c3 = ([120 230 180]+128)/(256+128);patch([0 1 1 0],[0 0 1 1],c1);patch([0 1 1 1-e 1-e 0+e],[0 0 1 1-e 0+e 0+e],c2);patch([0 0 1 1-e 0+e 0+e],[0 1 1 1-e 1-e 0+e],c3);plot([0 1 1 0 0],[0 0 1 1 0]);
  wires:
  "a{1} "/1 -> Delays 1/1("p{2}")
  Delays 1/1("pd{2,1}") -> "LW{2,1}"/1("ad{2,1}")
  "LW{2,1}"/1("lz{2,1}") -> netsum/1
  "b{2}"/1 -> netsum/2
  netsum/1 -> purelin/1
  purelin/1 -> "a{2}"/1

== system Control_planta_no_lineal_y_NN_mejor/MLP 10 14400/Function Fitting Neural Network1/Process Input 1 ==
  x : Inport  PortDimensions=11
      mask Display: e = 0.06;c1 = [120 230 180]/255;c2 = ([120 230 180]+0)/(256+128);c3 = ([120 230 180]+128)/(256+128);patch([0 1 1 0],[0 0 1 1],c1);patch([0 1 1 1-e 1-e 0+e],[0 0 1 1-e 0+e 0+e],c2);patch([0 0 1 1-e 0+e 0+e],[0 1 1 1-e 1-e 0+e],c3);plot([0 1 1 0 0],[0 0 1 1 0]);
  p : Outport  PortDimensions=11
      mask Display: e = 0.06;c1 = [120 230 180]/255;c2 = ([120 230 180]+0)/(256+128);c3 = ([120 230 180]+128)/(256+128);patch([0 1 1 0],[0 0 1 1],c1);patch([0 1 1 1-e 1-e 0+e],[0 0 1 1-e 0+e 0+e],c2);patch([0 0 1 1-e 0+e 0+e],[0 1 1 1-e 1-e 0+e],c3);plot([0 1 1 0 0],[0 0 1 1 0]);
  wires:
  x/1 -> p/1

== system Control_planta_no_lineal_y_NN_mejor/MLP 10 14400/Function Fitting Neural Network1/Process Output 1 ==
  a : Inport  PortDimensions=1
      mask Display: e = 0.06;c1 = [120 230 180]/255;c2 = ([120 230 180]+0)/(256+128);c3 = ([120 230 180]+128)/(256+128);patch([0 1 1 0],[0 0 1 1],c1);patch([0 1 1 1-e 1-e 0+e],[0 0 1 1-e 0+e 0+e],c2);patch([0 0 1 1-e 0+e 0+e],[0 1 1 1-e 1-e 0+e],c3);plot([0 1 1 0 0],[0 0 1 1 0]);
  y : Outport  PortDimensions=1
      mask Display: e = 0.06;c1 = [120 230 180]/255;c2 = ([120 230 180]+0)/(256+128);c3 = ([120 230 180]+128)/(256+128);patch([0 1 1 0],[0 0 1 1],c1);patch([0 1 1 1-e 1-e 0+e],[0 0 1 1-e 0+e 0+e],c2);patch([0 0 1 1-e 0+e 0+e],[0 1 1 1-e 1-e 0+e],c3);plot([0 1 1 0 0],[0 0 1 1 0]);
  wires:
  a/1 -> y/1

== system Control_planta_no_lineal_y_NN_mejor/MLP 10 3600/Function Fitting Neural Network/Layer 1 ==
  "p{1}" : Inport  PortDimensions=11
      mask Display: e = 0.06;c1 = [120 230 180]/255;c2 = ([120 230 180]+0)/(256+128);c3 = ([120 230 180]+128)/(256+128);patch([0 1 1 0],[0 0 1 1],c1);patch([0 1 1 1-e 1-e 0+e],[0 0 1 1-e 0+e 0+e],c2);patch([0 0 1 1-e 0+e 0+e],[0 1 1 1-e 1-e 0+e],c3);plot([0 1 1 0 0],[0 0 1 1 0]);
  Delays 1 : Subsystem
      mask Display: e = 0.06;c1 = [120 150 230]/255;c2 = ([120 150 230]+0)/383;c3 = ([120 150 230]+128)/383;patch([0 1 1 0],[0 0 1 1],c1);patch([0 1 1 1-e 1-e 0+e],[0 0 1 1-e 0+e 0+e],c2);patch([0 0 1 1-e 0+e 0+e],[0 1 1 1-e 1-e 0+e],c3);plot([0 1 1 0 0],[0 0 1 1 0]);disp('0');
  "IW{1,1}" : Subsystem
      mask Display: e = 0.06;c1 = [120 150 230]/255;c2 = ([120 150 230]+0)/383;c3 = ([120 150 230]+128)/383;patch([0 1 1 0],[0 0 1 1],c1);patch([0 1 1 1-e 1-e 0+e],[0 0 1 1-e 0+e 0+e],c2);patch([0 0 1 1-e 0+e 0+e],[0 1 1 1-e 1-e 0+e],c3);plot([0 1 1 0 0],[0 0 1 1 0]);disp('W');
  "b{1}" : Constant  Value=[-2.15522235861495925490771696786396205425262451171875;-1.704275208046103440295837572193704545497894287109375;-2.676572574208414767582553395186550915241241455078125;1.6645579111374597669481545381131581962108612060546875;0.06783136764068618818068756581851630471646785736083984375;-0.477579440029956725499715730620664544403553009033203125;1.766037536843283906051738085807301104068756103515625;1.032800638643438961850051782676018774509429931640625;-2.4601673059140285459989172522909939289093017578125;-1.614531194988896967146274619153700768947601318359375]
      mask Display: e = 0.06;c1 = [120 150 230]/255;c2 = ([120 150 230]+0)/383;c3 = ([120 150 230]+128)/383;patch([0 1 1 0],[0 0 1 1],c1);patch([0 1 1 1-e 1-e 0+e],[0 0 1 1-e 0+e 0+e],c2);patch([0 0 1 1-e 0+e 0+e],[0 1 1 1-e 1-e 0+e],c3);plot([0 1 1 0 0],[0 0 1 1 0]);disp('b');
  netsum : Sum  Inputs=2  InputSameDT=on  SaturateOnIntegerOverflow=on  OutDataTypeStr=Inherit: Same as first input
      mask Display: e = 0.06;c1 = [120 150 230]/255;c2 = ([120 150 230]+0)/383;c3 = ([120 150 230]+128)/383;patch([0 1 1 0],[0 0 1 1],c1);patch([0 1 1 1-e 1-e 0+e],[0 0 1 1-e 0+e 0+e],c2);patch([0 0 1 1-e 0+e 0+e],[0 1 1 1-e 1-e 0+e],c3);plot([0 1 1 0 0],[0 0 1 1 0]);disp('+');
  tansig : neural/Transfer Functions/tansig
  "a{1}" : Outport  InitialOutput=[0;0;0;0;0;0;0;0;0;0]
      mask Display: e = 0.06;c1 = [120 230 180]/255;c2 = ([120 230 180]+0)/(256+128);c3 = ([120 230 180]+128)/(256+128);patch([0 1 1 0],[0 0 1 1],c1);patch([0 1 1 1-e 1-e 0+e],[0 0 1 1-e 0+e 0+e],c2);patch([0 0 1 1-e 0+e 0+e],[0 1 1 1-e 1-e 0+e],c3);plot([0 1 1 0 0],[0 0 1 1 0]);
  wires:
  "p{1}"/1 -> Delays 1/1("p{1}")
  Delays 1/1("pd{1,1}") -> "IW{1,1}"/1("pd{1,1}")
  "IW{1,1}"/1("iz{1,1}") -> netsum/1
  "b{1}"/1 -> netsum/2
  netsum/1 -> tansig/1
  tansig/1 -> "a{1}"/1
